simulink model "MMMS_v3"  (R2024b)
settings: Solver=VariableStepAuto  StartTime=0.0  StopTime=60  FixedStep=0.001  RelTol=1e-3
InitFcn:
  | %rho_0t=[0.29;0.29;0.29]; %m
  | %V_0t=[-0.001;-0.001;0];%[-0.0005;-0.0005;0];
  | %w_t=[0;0;-0.002];
  | 
  | 
  | %rho_0t=[0.3;0.3;0.2]; %m
  | %V_0t=[-0.001;-0.001;0];%[-0.0005;-0.0005;0];
  | %w_t=[0;0;-0.001];
values from neighbouring files (symbols this model uses):
  Dt = 0.1    [main_EKF.m]
  Fake_Manip_grad = -0.2.*eye(7)    [Initiate_FQ.m]
  g_cm = zeros(4,4,n)    [Initiate_KUKA_inv.m]    (also in Main_MMMS.m; test_KUKA_elements.m)
  g_It00 = [eye(3) rho_It;0 0 0 1]    [main_EKF.m]
  iota0 = eye(6,6)    [Initiate_KUKA_inv.m]    (also in Main_MMMS.m; test_KUKA_elements.m)
  K_d = 10*[1.3*eye(3) zeros(3);zeros(3) 0.8*eye(3)]    [Initiate_FQ.m]    (also in Initiate_KUKA_inv.m = 5*[0.7*eye(3) zeros(3);zeros(3) 0.5*eye(3)]; MMMS_Initiate_FQ.m; Main_MMMS.m = 5*[0.7*eye(3) zeros(3);zeros(3) 0.5*eye(3)]; test_KUKA_elements.m = 50*[0.7*eye(3) zeros(3);zeros(3) 0.5*eye(3)])
  K_i = 5*[0.1*eye(3) zeros(3);zeros(3) 0.01*eye(3)]    [Initiate_FQ.m]    (also in Initiate_KUKA_inv.m = 5*[0.01*eye(3) zeros(3);zeros(3) 0.001*eye(3)]; MMMS_Initiate_FQ.m; Main_MMMS.m = 5*[0.01*eye(3) zeros(3);zeros(3) 0.001*eye(3)]; test_KUKA_elements.m = 50*[0.01*eye(3) zeros(3);zeros(3) 0.001*eye(3)])
  K_p = 100*[0.1 0 0 0 0 0;0 0.1 0 0 0 0; 0 0 0.1 0 0 0; 0 0 0 0.01 0 0 ... (first row only)    [Initiate_FQ.m]    (also in Initiate_KUKA_inv.m = 5*[0.1 0 0 0 0 0;0 0.1 0 0 0 0; 0 0 0.1 0 0 0; 0 0 0 0.01 0 ; MMMS_Initiate_FQ.m; Main_MMMS.m = 5*[0.1 0 0 0 0 0;0 0.1 0 0 0 0; 0 0 0.1 0 0 0; 0 0 0 0.01 0 ; test_KUKA_elements.m = 50*[0.1 0 0 0 0 0;0 0.1 0 0 0 0; 0 0 0.1 0 0 0; 0 0 0 0.01 0)
  K_w = 200*eye(7)    [Initiate_FQ.m]    (also in MMMS_Initiate_FQ.m)
  K_wd = 2*eye(7)    [Initiate_FQ.m]    (also in MMMS_Initiate_FQ.m)
  m = randn(s,total_time_steps,6)*chol(R)    [main_EKF.m]
  M0 = M_temp.M0.data(:,:,1)    [Initiate_FQ.m]    (also in MMMS_Initiate_FQ.m; test_KUKA_elements.m)
  m0 = robot.Bodies{1,n+1}.Mass    [Initiate_KUKA_inv.m]    (also in Main_MMMS.m; test_KUKA_elements.m)
  m0_frak = diag_M(1:6,1:6)    [Initiate_KUKA_inv.m]    (also in Main_MMMS.m; make_uncertain.m = diag_M_unc(1:6,1:6); test_KUKA_elements.m)
  M0m = M_temp.M0m.data(:,:,1)    [Initiate_FQ.m]    (also in MMMS_Initiate_FQ.m; test_KUKA_elements.m)
  m_diag = diag_M(7:end,7:end)    [Initiate_KUKA_inv.m]    (also in Main_MMMS.m; make_uncertain.m = diag_M_unc(7:end,7:end); test_KUKA_elements.m)
  M_t = (((Adjoint(g_It))'\M_t_body)/(Adjoint(g_It)))    [Initiate_FQ.m]    (also in Initiate_KUKA_inv.m = [eye(3)*mt zeros(3); zeros(3) eye(3)*80]; MMMS_Initiate_FQ.m; Main_MMMS.m = [eye(3)*mt zeros(3); zeros(3) eye(3)*80]; test_KUKA_elements.m = [eye(3)*mt zeros(3); zeros(3) eye(3)*80])
  M_t_body = [eye(3)*mt zeros(3); zeros(3) eye(3)*0.416667]    [Initiate_FQ.m]    (also in MMMS_Initiate_FQ.m)
  mm = zeros(1,n)    [Initiate_KUKA_inv.m]    (also in Main_MMMS.m; test_KUKA_elements.m)
  mu = P0    [Initiate_FQ.m]    (also in Initiate_KUKA_inv.m = zeros(6,1); MMMS_Initiate_FQ.m; Main_MMMS.m = zeros(6,1); make_uncertain.m = P0_unc)
  mu_t = inv((Adjoint(g_It))')*M_t_body*[V_It;w_t]    [Initiate_FQ.m]    (also in Initiate_KUKA_inv.m = M_t*[V_0t;w_t]; MMMS_Initiate_FQ.m; Main_MMMS.m = M_t*[V_0t;w_t]; make_uncertain.m = inv((Adjoint(g_It))')*M_t_body_unc*[V_It;w_t])
  noise_st = 0.000005    (= 5e-06)    [main_EKF.m]
  q_dot_m = [0;0;0;0;0;0;0]    [Initiate_FQ.m]    (also in Initiate_KUKA_inv.m; MMMS_Initiate_FQ.m; Main_MMMS.m; test_KUKA_elements.m = [0])
  q_m = [0.2;1.2;0.3;2.5;0.5;1.5;0.6]    [Initiate_FQ.m]    (also in Initiate_KUKA_inv.m = [0;0;0;0;0;0;0]; MMMS_Initiate_FQ.m = [0.2;0.2;0.3;0.5;0.5;0.5;0.6]; Main_MMMS.m = [0;0;0;0;0;0;0]; test_KUKA_elements.m = [0.2;1.2;0.3;1.8;0.5;1.3;0.6])
  rho_It = [0;0;1.7]    [Initiate_FQ.m]    (also in MMMS_Initiate_FQ.m)
  s = RandStream.create('mrg32k3a','NumStreams',1)    [main_EKF.m]
  sc_size = 1    [Initiate_KUKA_inv.m]    (also in Main_MMMS.m; test_KUKA_elements.m)
  V_It = [0.0005;0.0005;0]    [Initiate_FQ.m]    (also in MMMS_Initiate_FQ.m = [0.001;0.001;0])
  Xi_m_matrix = zeros(6*n,n)    [Initiate_KUKA_inv.m]    (also in Main_MMMS.m)
undefined symbols (not defined in the file or in its folder): g_cm0, I0, Im, Mm, X, Xi_m, Y, Z
libraries: nesl_utility x314, sm_lib x231, robotcorelib x30, simulink x12
(part 3 of 13)

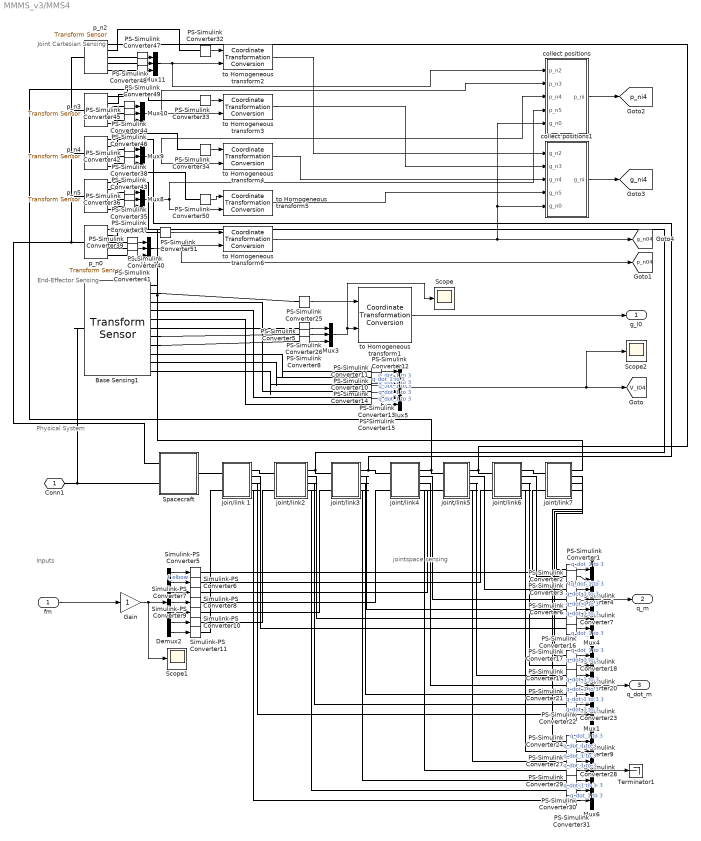
== system MMMS_v3/MMS4 ==
  note: Joint Cartesian Sensing
  note: End-Effector Sensing
  note: Inputs
  note: jointspace sensing
  note: Physical System
  fm : Inport
  Base Sensing1 : sm_lib/Frames and Transforms/Transform Sensor  MeasurementFrame=NonRotatingBase  RotationSequence=XYZ  SenseAngle=off  SenseAxis=off  SenseQ=off  SenseR=on  SenseRotationSequence=off  SenseOmegaX=on  SenseOmegaY=on  SenseOmegaZ=on  SenseOmega=off  SenseQDot=off  SenseRDot=off  SenseRotationSequenceDot=off  SenseAlphaX=off  SenseAlphaY=off  SenseAlphaZ=off  SenseAlpha=off  SenseQDDot=off  SenseRDDot=off  SenseX=on  SenseY=on  SenseZ=on  SenseXYZ=off  SenseRad=off  SenseAzim=off  SenseDist=off  SenseInc=off  SenseXDot=on  SenseYDot=on  SenseZDot=on  SenseXYZDot=off  SenseRadDot=off  SenseAzimDot=off  SenseDistDot=off  SenseIncDot=off  SenseXDDot=off  SenseYDDot=off  SenseZDDot=off  SenseXYZDDot=off  SenseRadDDot=off  SenseAzimDDot=off  SenseDistDDot=off  SenseIncDDot=off
  Demux2 : Demux  Outputs=7
  Gain : Gain
  Mux1 : Mux  Inputs=7
  Mux{2..3,8..11} (6 alike) : Mux  Inputs=3
  Mux4 : Mux  Inputs=7
  Mux5 : Mux  Inputs=6
  Mux6 : Mux  Inputs=7
  PS-Simulink Converter{1..51} (51 alike) : nesl_utility/PS-Simulink Converter  PhysicalDomain=network_engine_domain  SubClassName=ps_output  LeftPortType=input  RightPortType=output  PseudoPeriodic=off  Frequencies=[]  VectorFormat=1-D array  Unit=inherit  AffineConversion=off
  Scope : Scope
  Scope1 : Scope
  Scope2 : Scope
  Simulink-PS Converter{5..11} (7 alike) : nesl_utility/Simulink-PS Converter  PhysicalDomain=network_engine_domain  SubClassName=ps_input  LeftPortType=input  RightPortType=output  PseudoPeriodic=off  Frequencies=[]  NoiseDistribution=none  NoiseParameters=[]  Unit=1  AffineConversion=off  FilteringAndDerivatives=provide  SimscapeFilterOrder=1  InputFilterTimeConstant=0.001  UdotUserProvided=0
  Spacecraft : Subsystem
  Terminator1 : Terminator
  collect positions : MATLAB Function  TreatAsAtomicUnit=on
  collect positions1 : MATLAB Function  TreatAsAtomicUnit=on
  join/link 1 : Subsystem
  joint/link2 : Subsystem
  joint/link3 : Subsystem
  joint/link4 : Subsystem
  joint/link5 : Subsystem
  joint/link6 : Subsystem
  joint/link7 : Subsystem
  p_n{0,2..5} (5 alike) : sm_lib/Frames and Transforms/Transform Sensor  MeasurementFrame=Base  RotationSequence=XYZ  SenseAngle=off  SenseAxis=off  SenseQ=off  SenseR=on  SenseRotationSequence=off  SenseOmegaX=off  SenseOmegaY=off  SenseOmegaZ=off  SenseOmega=off  SenseQDot=off  SenseRDot=off  SenseRotationSequenceDot=off  SenseAlphaX=off  SenseAlphaY=off  SenseAlphaZ=off  SenseAlpha=off  SenseQDDot=off  SenseRDDot=off  SenseX=on  SenseY=on  SenseZ=on  SenseXYZ=off  SenseRad=off  SenseAzim=off  SenseDist=off  SenseInc=off  SenseXDot=off  SenseYDot=off  SenseZDot=off  SenseXYZDot=off  SenseRadDot=off  SenseAzimDot=off  SenseDistDot=off  SenseIncDot=off  SenseXDDot=off  SenseYDDot=off  SenseZDDot=off  SenseXYZDDot=off  SenseRadDDot=off  SenseAzimDDot=off  SenseDistDDot=off  SenseIncDDot=off
  to Homogeneous transform{1..6} (6 alike) : robotcorelib/Coordinate Transformation Conversion  InputRepresentation=Rotation Matrix  InputEulerSequence=ZYX  ShowTrVecInputPort=on  OutputRepresentation=Homogeneous Transformation  OutputEulerSequence=ZYX  ShowTrVecOutputPort=on  SimulateUsing=Code generation
  Conn1 : PMIOPort  Side=Left
  g_I0 : Outport
  q_m : Outport  Port=2
  q_dot_m : Outport  Port=3
  tag scope: V_I04=global, g_n04=global, g_ni4=global, p_n04=global, p_ni4=global
  wires:
  to Homogeneous transform5/1 -> collect positions1/4(g_n5)
  to Homogeneous transform4/1 -> collect positions1/3(g_n4)
  to Homogeneous transform3/1 -> collect positions1/2(g_n3)
  to Homogeneous transform2/1 -> collect positions1/1(g_n2)
  to Homogeneous transform6/1 -> [g_n04], collect positions1/5(g_n0), collect positions/5(g_n0)
  PS-Simulink Converter51/1 -> to Homogeneous transform6/1
  collect positions1/1(g_ni) -> [g_ni4]
  Mux8/1 -> collect positions/4(p_n5), to Homogeneous transform5/2
  PS-Simulink Converter50/1 -> to Homogeneous transform5/1
  PS-Simulink Converter34/1 -> to Homogeneous transform4/1
  Mux9/1 -> collect positions/3(p_n4), to Homogeneous transform4/2
  Mux10/1 -> collect positions/2(p_n3), to Homogeneous transform3/2
  PS-Simulink Converter33/1 -> to Homogeneous transform3/1
  PS-Simulink Converter32/1 -> to Homogeneous transform2/1
  collect positions/1(p_ni) -> [p_ni4]
  PS-Simulink Converter49/1 -> Mux11/3
  PS-Simulink Converter47/1 -> Mux11/1
  PS-Simulink Converter48/1 -> Mux11/2
  Mux11/1 -> collect positions/1(p_n2), to Homogeneous transform2/2
  PS-Simulink Converter46/1 -> Mux10/3
  PS-Simulink Converter44/1 -> Mux10/1
  PS-Simulink Converter45/1 -> Mux10/2
  PS-Simulink Converter43/1 -> Mux9/3
  PS-Simulink Converter38/1 -> Mux9/1
  PS-Simulink Converter42/1 -> Mux9/2
  PS-Simulink Converter37/1 -> Mux8/3
  PS-Simulink Converter35/1 -> Mux8/1
  PS-Simulink Converter36/1 -> Mux8/2
  PS-Simulink Converter41/1 -> Mux2/3
  PS-Simulink Converter40/1 -> Mux2/2
  PS-Simulink Converter39/1 -> Mux2/1
  Mux2/1 -> [p_n04], to Homogeneous transform6/2
  Mux5/1 -> Scope2/1, [V_I04]
  PS-Simulink Converter19/1 -> Mux1/3  "q_dot_1 to 3"
  PS-Simulink Converter17/1 -> Mux1/1  "q_dot_1 to 3"
  PS-Simulink Converter22/1 -> Mux1/6  "q_dot_1 to 3"
  PS-Simulink Converter29/1 -> Mux6/5  "q_dot_1 to 3"
  PS-Simulink Converter20/1 -> Mux1/4  "q_dot_1 to 3"
  Mux6/1 -> Terminator1/1
  PS-Simulink Converter24/1 -> Mux6/1  "q_dot_1 to 3"
  Mux1/1 -> q_dot_m/1
  Mux4/1 -> q_m/1
  PS-Simulink Converter28/1 -> Mux6/4  "q_dot_1 to 3"
  PS-Simulink Converter16/1 -> Mux4/7  "q_dot_1 to 3"
  PS-Simulink Converter23/1 -> Mux1/7  "q_dot_1 to 3"
  PS-Simulink Converter21/1 -> Mux1/5  "q_dot_1 to 3"
  PS-Simulink Converter4/1 -> Mux4/4  "q_dot_1 to 3"
  PS-Simulink Converter2/1 -> Mux4/2  "q_dot_1 to 3"
  PS-Simulink Converter7/1 -> Mux4/6  "q_dot_1 to 3"
  PS-Simulink Converter9/1 -> Mux6/2  "q_dot_1 to 3"
  PS-Simulink Converter31/1 -> Mux6/7  "q_dot_1 to 3"
  PS-Simulink Converter18/1 -> Mux1/2  "q_dot_1 to 3"
  PS-Simulink Converter3/1 -> Mux4/3  "q_dot_1 to 3"
  PS-Simulink Converter30/1 -> Mux6/6  "q_dot_1 to 3"
  PS-Simulink Converter6/1 -> Mux4/5  "q_dot_1 to 3"
  PS-Simulink Converter1/1 -> Mux4/1  "q_dot_1 to 3"
  PS-Simulink Converter27/1 -> Mux6/3  "q_dot_1 to 3"
  Demux2/5 -> Simulink-PS Converter9/1
  Demux2/2 -> Simulink-PS Converter6/1  "f_elbow"
  Demux2/6 -> Simulink-PS Converter10/1
  PS-Simulink Converter5/1 -> Mux3/2
  PS-Simulink Converter11/1 -> Mux5/1  "q_dot_1 to 3"
  Demux2/4 -> Simulink-PS Converter8/1
  PS-Simulink Converter14/1 -> Mux5/5  "q_dot_1 to 3"
  Demux2/7 -> Simulink-PS Converter11/1
  PS-Simulink Converter26/1 -> Mux3/1
  PS-Simulink Converter13/1 -> Mux5/4  "q_dot_1 to 3"
  to Homogeneous transform1/1 -> g_I0/1
  PS-Simulink Converter12/1 -> Mux5/2  "q_dot_1 to 3"
  Mux3/1 -> to Homogeneous transform1/2, Scope/1
  PS-Simulink Converter8/1 -> Mux3/3
  Gain/1 -> Demux2/1, Scope1/1
  PS-Simulink Converter25/1 -> to Homogeneous transform1/1
  fm/1 -> Gain/1
  PS-Simulink Converter10/1 -> Mux5/3  "q_dot_1 to 3"
  PS-Simulink Converter15/1 -> Mux5/6  "q_dot_1 to 3"
  Demux2/3 -> Simulink-PS Converter7/1
  Demux2/1 -> Simulink-PS Converter5/1
  connections:
  p_n0/RConn2 -- PS-Simulink Converter51/LConn1
  p_n5/RConn2 -- PS-Simulink Converter50/LConn1
  p_n4/RConn2 -- PS-Simulink Converter34/LConn1
  p_n3/RConn2 -- PS-Simulink Converter33/LConn1
  PS-Simulink Converter32/LConn1 -- p_n2/RConn2
  p_n2/RConn4 -- PS-Simulink Converter48/LConn1
  p_n2/RConn3 -- PS-Simulink Converter47/LConn1
  PS-Simulink Converter49/LConn1 -- p_n2/RConn5
  p_n3/RConn4 -- PS-Simulink Converter45/LConn1
  p_n3/RConn3 -- PS-Simulink Converter44/LConn1
  PS-Simulink Converter46/LConn1 -- p_n3/RConn5
  p_n4/RConn4 -- PS-Simulink Converter42/LConn1
  p_n4/RConn3 -- PS-Simulink Converter38/LConn1
  PS-Simulink Converter43/LConn1 -- p_n4/RConn5
  p_n5/RConn4 -- PS-Simulink Converter36/LConn1
  p_n5/RConn3 -- PS-Simulink Converter35/LConn1
  PS-Simulink Converter37/LConn1 -- p_n5/RConn5
  p_n0/RConn3 -- PS-Simulink Converter39/LConn1
  p_n0/LConn1 -- p_n5/LConn1 -- p_n4/LConn1 -- p_n3/LConn1 -- p_n2/LConn1 -- Spacecraft/LConn1
  p_n0/RConn4 -- PS-Simulink Converter40/LConn1
  PS-Simulink Converter41/LConn1 -- p_n0/RConn5
  join/link 1/RConn3 -- PS-Simulink Converter23/LConn1
  joint/link2/RConn3 -- PS-Simulink Converter22/LConn1
  join/link 1/RConn4 -- PS-Simulink Converter31/LConn1
  joint/link2/RConn4 -- PS-Simulink Converter30/LConn1
  PS-Simulink Converter7/LConn1 -- joint/link2/RConn2
  join/link 1/RConn2 -- PS-Simulink Converter16/LConn1
  joint/link2/RConn1 -- p_n5/RConn1 -- joint/link3/LConn1
  Simulink-PS Converter10/RConn1 -- joint/link2/LConn2
  join/link 1/RConn1 -- joint/link2/LConn1
  join/link 1/LConn1 -- Spacecraft/RConn1
  join/link 1/LConn2 -- Simulink-PS Converter11/RConn1
  joint/link7/RConn4 -- PS-Simulink Converter24/LConn1
  joint/link7/RConn3 -- PS-Simulink Converter17/LConn1
  joint/link7/RConn2 -- PS-Simulink Converter1/LConn1
  joint/link6/LConn2 -- Simulink-PS Converter6/RConn1
  joint/link6/RConn2 -- PS-Simulink Converter2/LConn1
  joint/link6/RConn1 -- joint/link7/LConn1
  joint/link3/RConn4 -- PS-Simulink Converter29/LConn1
  joint/link3/RConn3 -- PS-Simulink Converter21/LConn1
  joint/link3/RConn2 -- PS-Simulink Converter6/LConn1
  joint/link4/RConn4 -- PS-Simulink Converter28/LConn1
  joint/link4/RConn3 -- PS-Simulink Converter20/LConn1
  joint/link4/RConn2 -- PS-Simulink Converter4/LConn1
  joint/link5/RConn4 -- PS-Simulink Converter27/LConn1
  joint/link5/RConn3 -- PS-Simulink Converter19/LConn1
  joint/link5/RConn2 -- PS-Simulink Converter3/LConn1
  joint/link6/RConn4 -- PS-Simulink Converter9/LConn1
  joint/link6/RConn3 -- PS-Simulink Converter18/LConn1
  Simulink-PS Converter7/RConn1 -- joint/link5/LConn2
  Base Sensing1/RConn6 -- PS-Simulink Converter26/LConn1
  Base Sensing1/RConn8 -- PS-Simulink Converter8/LConn1
  Base Sensing1/RConn9 -- PS-Simulink Converter11/LConn1
  Base Sensing1/RConn4 -- PS-Simulink Converter14/LConn1
  Simulink-PS Converter5/RConn1 -- joint/link7/LConn2
  Base Sensing1/RConn3 -- PS-Simulink Converter13/LConn1
  Base Sensing1/RConn11 -- PS-Simulink Converter10/LConn1
  p_n2/RConn1 -- joint/link5/RConn1 -- joint/link6/LConn1
  Base Sensing1/RConn7 -- PS-Simulink Converter5/LConn1
  Base Sensing1/RConn5 -- PS-Simulink Converter15/LConn1
  p_n3/RConn1 -- joint/link4/RConn1 -- joint/link5/LConn1
  Base Sensing1/RConn2 -- PS-Simulink Converter25/LConn1
  Simulink-PS Converter8/RConn1 -- joint/link4/LConn2
  Simulink-PS Converter9/RConn1 -- joint/link3/LConn2
  Base Sensing1/RConn10 -- PS-Simulink Converter12/LConn1
  joint/link3/RConn1 -- p_n4/RConn1 -- joint/link4/LConn1
  joint/link7/RConn1 -- Base Sensing1/RConn1 -- p_n0/RConn1
  Base Sensing1/LConn1 -- Spacecraft/LConn2 -- Conn1/RConn1

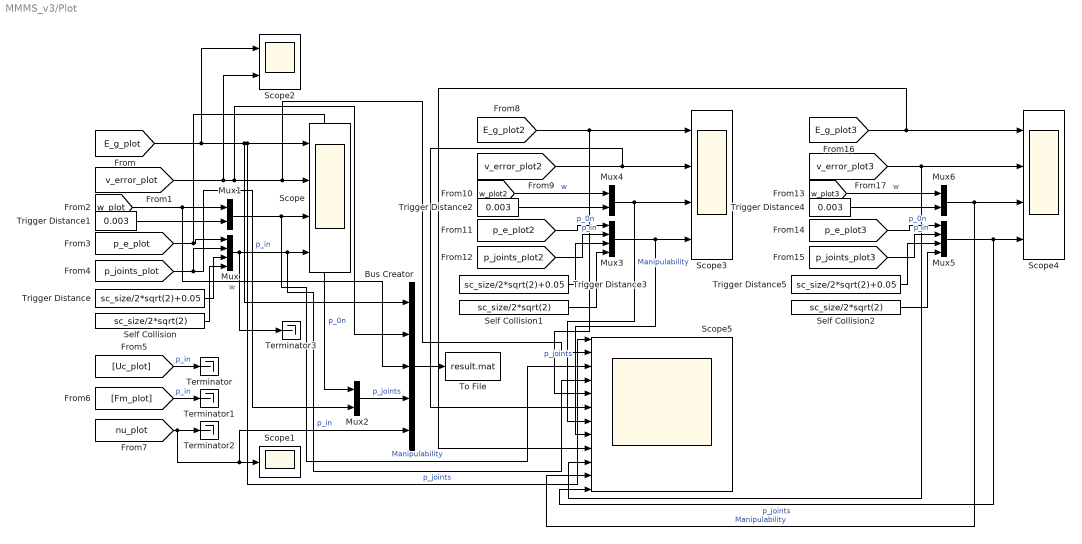
== system MMMS_v3/Plot ==
  Bus Creator : BusCreator  Inputs=5
  Mux : Mux  Inputs=[1 4 1 1]
  Mux{1..2,4,6} (4 alike) : Mux  Inputs=2
  Mux3 : Mux  Inputs=[1 4 1 1]
  Mux5 : Mux  Inputs=[1 4 1 1]
  Scope : Scope  NumInputPorts=4
  Scope1 : Scope
  Scope2 : Scope  NumInputPorts=2
  Scope3 : Scope  NumInputPorts=4
  Scope4 : Scope  NumInputPorts=4
  Scope5 : Scope  NumInputPorts=12
  Self Collision : Constant  Value=sc_size/2*sqrt(2)
  Self Collision1 : Constant  Value=sc_size/2*sqrt(2)
  Self Collision2 : Constant  Value=sc_size/2*sqrt(2)
  Terminator{,1..3} (4 alike) : Terminator
  To File : ToFile  Filename=result.mat
  Trigger Distance : Constant  Value=sc_size/2*sqrt(2)+0.05
  Trigger Distance1 : Constant  Value=0.003
  Trigger Distance2 : Constant  Value=0.003
  Trigger Distance3 : Constant  Value=sc_size/2*sqrt(2)+0.05
  Trigger Distance4 : Constant  Value=0.003
  Trigger Distance5 : Constant  Value=sc_size/2*sqrt(2)+0.05
  wires:
  [E_g_plot] -> Scope2/1, Bus Creator/1, Scope/1, Scope5/1
  [v_error_plot] -> Scope2/2, Bus Creator/2, Scope5/2, Scope/2
  [w_plot] -> Bus Creator/3, Mux1/1  "w"
  [p_e_plot] -> Mux2/1, Mux/1  "p_0n"
  [p_joints_plot] -> Mux/2, Mux2/2  "p_in"
  Mux/1 -> Scope5/4, Scope/4, Terminator3/1  "p_joints"
  Trigger Distance/1 -> Mux/3
  [Uc_plot] -> Terminator/1  "p_in"
  [Fm_plot] -> Terminator1/1  "p_in"
  [nu_plot] -> Bus Creator/5, Scope1/1, Terminator2/1  "p_in"
  Self Collision/1 -> Mux/4
  Trigger Distance1/1 -> Mux1/2
  Mux1/1 -> Scope5/3, Scope/3  "Manipulability"
  Bus Creator/1 -> To File/1
  Mux2/1 -> Bus Creator/4  "p_joints"
  [w_plot2] -> Mux4/1  "w"
  [v_error_plot2] -> Scope5/6, Scope3/2
  [p_joints_plot2] -> Mux3/2  "p_in"
  [E_g_plot2] -> Scope5/5, Scope3/1
  Trigger Distance2/1 -> Mux4/2
  Mux3/1 -> Scope5/8, Scope3/4  "p_joints"
  [p_e_plot2] -> Mux3/1  "p_0n"
  Mux4/1 -> Scope5/7, Scope3/3  "Manipulability"
  Trigger Distance3/1 -> Mux3/3
  Self Collision1/1 -> Mux3/4
  [p_joints_plot3] -> Mux5/2  "p_in"
  Trigger Distance5/1 -> Mux5/3
  Mux6/1 -> Scope5/11, Scope4/3  "Manipulability"
  Trigger Distance4/1 -> Mux6/2
  Mux5/1 -> Scope5/12, Scope4/4  "p_joints"
  [v_error_plot3] -> Scope5/10, Scope4/2
  [E_g_plot3] -> Scope5/9, Scope4/1
  [p_e_plot3] -> Mux5/1  "p_0n"
  Self Collision2/1 -> Mux5/4
  [w_plot3] -> Mux6/1  "w"

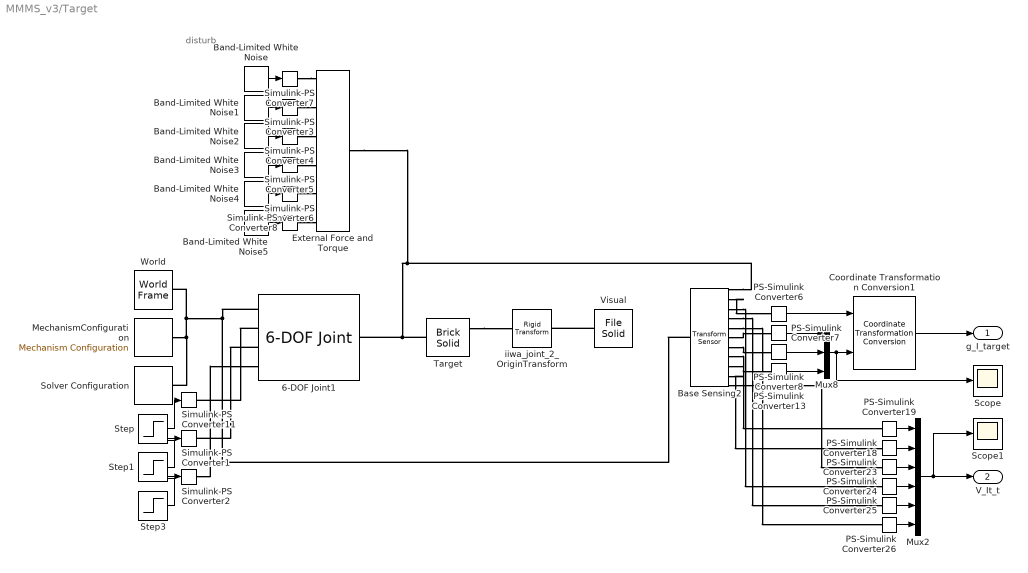
== system MMMS_v3/Target ==
  note: disturb
  6-DOF Joint1 : sm_lib/Joints/6-DOF Joint  JointMode=Normal  CompositeWrenchDir=FollowerOnBase  CompositeWrenchFrame=BaseFrame  SenseConstraintForce=off  SenseConstraintTorque=off  SenseTotalForce=off  SenseTotalTorque=off  PxPositionTargetSpecify=on  PxPositionTargetPriority=High  PxPositionTargetValue=rho_It(1)  PxPositionTargetValueUnits=m  PxVelocityTargetSpecify=on  PxVelocityTargetPriority=High  PxVelocityTargetValue=V_It(1)  PxVelocityTargetValueUnits=m/s  PxEquilibriumPosition=0  PxEquilibriumPositionUnits=m  PxSpringStiffness=0  PxSpringStiffnessUnits=N/m  PxDampingCoefficient=0  PxDampingCoefficientUnits=N/(m/s)  PxLowerLimitSpecify=off  PxLowerLimitBound=-1  PxLowerLimitBoundUnits=m  PxLowerLimitStiffness=1e6  PxLowerLimitStiffnessUnits=N/m  PxLowerLimitDamping=1e3  PxLowerLimitDampingUnits=N/(m/s)  PxLowerLimitTransitionRegionWidth=1e-4  PxLowerLimitTransitionRegionWidthUnits=m  PxUpperLimitSpecify=off  PxUpperLimitBound=1  PxUpperLimitBoundUnits=m  PxUpperLimitStiffness=1e6  PxUpperLimitStiffnessUnits=N/m  PxUpperLimitDamping=1e3  PxUpperLimitDampingUnits=N/(m/s)  PxUpperLimitTransitionRegionWidth=1e-4  PxUpperLimitTransitionRegionWidthUnits=m  PxTorqueActuationMode=InputTorque  PxMotionActuationMode=ComputedMotion  PxSensePosition=off  PxSenseVelocity=off  PxSenseAcceleration=off  PxSenseTorqueForce=off  PxSenseLowerLimitTorqueForce=off  PxSenseUpperLimitTorqueForce=off  PyPositionTargetSpecify=on  PyPositionTargetPriority=High  PyPositionTargetValue=rho_It(2)  PyPositionTargetValueUnits=m  PyVelocityTargetSpecify=on  PyVelocityTargetPriority=High  PyVelocityTargetValue=V_It(2)  PyVelocityTargetValueUnits=m/s  PyEquilibriumPosition=0  PyEquilibriumPositionUnits=m  PySpringStiffness=0  PySpringStiffnessUnits=N/m  PyDampingCoefficient=0  PyDampingCoefficientUnits=N/(m/s)  PyLowerLimitSpecify=off  PyLowerLimitBound=-1  PyLowerLimitBoundUnits=m  PyLowerLimitStiffness=1e6  PyLowerLimitStiffnessUnits=N/m  PyLowerLimitDamping=1e3  PyLowerLimitDampingUnits=N/(m/s)  PyLowerLimitTransitionRegionWidth=1e-4  PyLowerLimitTransitionRegionWidthUnits=m  PyUpperLimitSpecify=off  PyUpperLimitBound=1  PyUpperLimitBoundUnits=m  PyUpperLimitStiffness=1e6  PyUpperLimitStiffnessUnits=N/m  PyUpperLimitDamping=1e3  PyUpperLimitDampingUnits=N/(m/s)  PyUpperLimitTransitionRegionWidth=1e-4  PyUpperLimitTransitionRegionWidthUnits=m  PyTorqueActuationMode=InputTorque  PyMotionActuationMode=ComputedMotion  PySensePosition=off  PySenseVelocity=off  PySenseAcceleration=off  PySenseTorqueForce=off  PySenseLowerLimitTorqueForce=off  PySenseUpperLimitTorqueForce=off  PzPositionTargetSpecify=on  PzPositionTargetPriority=High  PzPositionTargetValue=rho_It(3)  PzPositionTargetValueUnits=m  PzVelocityTargetSpecify=on  PzVelocityTargetPriority=High  PzVelocityTargetValue=V_It(3)  PzVelocityTargetValueUnits=m/s  PzEquilibriumPosition=0  PzEquilibriumPositionUnits=m  PzSpringStiffness=0  PzSpringStiffnessUnits=N/m  PzDampingCoefficient=0  PzDampingCoefficientUnits=N/(m/s)  PzLowerLimitSpecify=off  PzLowerLimitBound=-1  PzLowerLimitBoundUnits=m  PzLowerLimitStiffness=1e6  PzLowerLimitStiffnessUnits=N/m  PzLowerLimitDamping=1e3  PzLowerLimitDampingUnits=N/(m/s)  PzLowerLimitTransitionRegionWidth=1e-4  PzLowerLimitTransitionRegionWidthUnits=m  PzUpperLimitSpecify=off  PzUpperLimitBound=1  PzUpperLimitBoundUnits=m  PzUpperLimitStiffness=1e6  PzUpperLimitStiffnessUnits=N/m  PzUpperLimitDamping=1e3  PzUpperLimitDampingUnits=N/(m/s)  PzUpperLimitTransitionRegionWidth=1e-4  PzUpperLimitTransitionRegionWidthUnits=m  PzTorqueActuationMode=InputTorque  PzMotionActuationMode=ComputedMotion  PzSensePosition=off  PzSenseVelocity=off  PzSenseAcceleration=off  PzSenseTorqueForce=off  PzSenseLowerLimitTorqueForce=off  PzSenseUpperLimitTorqueForce=off  SphPositionTargetSpecify=on  SphPositionTargetPriority=High  SphPositionTargetRotationMethod=RotationSequence  SphPositionTargetFollAlignAxisA=+X  SphPositionTargetBaseAlignAxisA=+Y  SphPositionTargetFollAlignAxisB=+Y  SphPositionTargetBaseAlignAxisB=+Z  SphPositionTargetRotationStandardAxis=+Z  SphPositionTargetRotationAngle=0.0  SphPositionTargetRotationAngleUnits=deg  SphPositionTargetRotationArbitraryAxis=[0 0 1]  SphPositionTargetRotationSequenceAxes=FollowerAxes  SphPositionTargetRotationSequence=XYZ  SphPositionTargetRotationSequenceAngles=[0 0 0]  SphPositionTargetRotationSequenceAnglesUnits=rad  SphPositionTargetRotationMatrix=[1 0 0; 0 1 0; 0 0 1]  SphPositionTargetQuaternion=[1 0 0 0]  SphVelocityTargetSpecify=on  SphVelocityTargetPriority=High  SphVelocityTargetValue=w_t  SphVelocityTargetValueUnits=rad/s  SphVelocityTargetInFollowerFrame=off  SphEqPosRotationMethod=None  SphEqPosFollAlignAxisA=+X  SphEqPosBaseAlignAxisA=+Y  SphEqPosFollAlignAxisB=+Y  SphEqPosBaseAlignAxisB=+Z  SphEqPosRotationStandardAxis=+Z  SphEqPosRotationAngle=0.0  SphEqPosRotationAngleUnits=deg  SphEqPosRotationArbitraryAxis=[0 0 1]  SphEqPosRotationSequenceAxes=FollowerAxes  SphEqPosRotationSequence=XYX  SphEqPosRotationSequenceAngles=[0 0 0]  SphEqPosRotationSequenceAnglesUnits=deg  SphEqPosRotationMatrix=[1 0 0; 0 1 0; 0 0 1]  SphEqPosQuaternion=[1 0 0 0]  SphSpringStiffness=0  SphSpringStiffnessUnits=N*m/deg  SphDampingCoefficient=0  SphDampingCoefficientUnits=N*m/(deg/s)  SphLowerLimitSpecify=off  SphLowerLimitBound=15  SphLowerLimitBoundUnits=deg  SphLowerLimitStiffness=1e4  SphLowerLimitStiffnessUnits=N*m/deg  SphLowerLimitDamping=10  SphLowerLimitDampingUnits=N*m/(deg/s)  SphLowerLimitTransitionRegionWidth=0.1  SphLowerLimitTransitionRegionWidthUnits=deg  SphUpperLimitSpecify=off  SphUpperLimitBound=45  SphUpperLimitBoundUnits=deg  SphUpperLimitStiffness=1e4  SphUpperLimitStiffnessUnits=N*m/deg  SphUpperLimitDamping=10  SphUpperLimitDampingUnits=N*m/(deg/s)  SphUpperLimitTransitionRegionWidth=0.1  SphUpperLimitTransitionRegionWidthUnits=deg  SphTorqueActuationMode=NoTorque  SphActuateTorqueX=off  SphActuateTorqueY=off  SphActuateTorqueZ=off  SphActuateTorque=off  SphActuationFrame=BaseFrame  SphSensePosition=off  SphSenseVelocityX=off  SphSenseVelocityY=off  SphSenseVelocityZ=off  SphSenseVelocity=off  SphSenseAccelerationX=off  SphSenseAccelerationY=off  SphSenseAccelerationZ=off  SphSenseAcceleration=off  SphSenseLowerLimitTorqueMag=off  SphSenseUpperLimitTorqueMag=off  SphSensingFrame=BaseFrame
  Band-Limited White Noise : simulink/Sources/Band-Limited White Noise  Cov=dist_force  Ts=0.1  seed=[23347]
  Band-Limited White Noise1 : simulink/Sources/Band-Limited White Noise  Cov=dist_force  Ts=0.1  seed=[23348]
  Band-Limited White Noise2 : simulink/Sources/Band-Limited White Noise  Cov=[0.0000001]  Ts=0.1  seed=[23343]
  Band-Limited White Noise3 : simulink/Sources/Band-Limited White Noise  Cov=dist_force  Ts=0.1  seed=[23342]
  Band-Limited White Noise4 : simulink/Sources/Band-Limited White Noise  Cov=dist_Force  Ts=0.1  seed=[23345]
  Band-Limited White Noise5 : simulink/Sources/Band-Limited White Noise  Cov=dist_force  Ts=0.1  seed=[23341]
  Base Sensing2 : sm_lib/Frames and Transforms/Transform Sensor  MeasurementFrame=NonRotatingBase  RotationSequence=XYZ  SenseAngle=off  SenseAxis=off  SenseQ=off  SenseR=on  SenseRotationSequence=off  SenseOmegaX=on  SenseOmegaY=on  SenseOmegaZ=on  SenseOmega=off  SenseQDot=off  SenseRDot=off  SenseRotationSequenceDot=off  SenseAlphaX=off  SenseAlphaY=off  SenseAlphaZ=off  SenseAlpha=off  SenseQDDot=off  SenseRDDot=off  SenseX=on  SenseY=on  SenseZ=on  SenseXYZ=off  SenseRad=off  SenseAzim=off  SenseDist=off  SenseInc=off  SenseXDot=on  SenseYDot=on  SenseZDot=on  SenseXYZDot=off  SenseRadDot=off  SenseAzimDot=off  SenseDistDot=off  SenseIncDot=off  SenseXDDot=off  SenseYDDot=off  SenseZDDot=off  SenseXYZDDot=off  SenseRadDDot=off  SenseAzimDDot=off  SenseDistDDot=off  SenseIncDDot=off
  Coordinate Transformation Conversion1 : robotcorelib/Coordinate Transformation Conversion  InputRepresentation=Rotation Matrix  InputEulerSequence=ZYX  ShowTrVecInputPort=on  OutputRepresentation=Homogeneous Transformation  OutputEulerSequence=ZYX  ShowTrVecOutputPort=on  SimulateUsing=Interpreted execution
  External Force and Torque : sm_lib/Forces and Torques/External Force and Torque  EnableForceX=on  EnableForceY=on  EnableForceZ=on  EnableForce=off  ForceResolutionFrame=AttachedFrame  EnableTorqueX=on  EnableTorqueY=on  EnableTorqueZ=on  EnableTorque=off  TorqueResolutionFrame=AttachedFrame
  MechanismConfiguration : sm_lib/Utilities/Mechanism Configuration  UniformGravity=Constant  GravityVector=[0 0 0]  GravityVectorUnits=m/s^2  LinearizationDelta=0.001  JointModeTransitionNonlinearIterations=2
  Mux2 : Mux  Inputs=6
  Mux8 : Mux  Inputs=3
  PS-Simulink Converter{6..8,13,18..19,23..26} (10 alike) : nesl_utility/PS-Simulink Converter  PhysicalDomain=network_engine_domain  SubClassName=ps_output  LeftPortType=input  RightPortType=output  PseudoPeriodic=off  Frequencies=[]  VectorFormat=1-D array  Unit=inherit  AffineConversion=off
  Scope : Scope
  Scope1 : Scope
  Simulink-PS Converter{1..8,11} (9 alike) : nesl_utility/Simulink-PS Converter  PhysicalDomain=network_engine_domain  SubClassName=ps_input  LeftPortType=input  RightPortType=output  PseudoPeriodic=off  Frequencies=[]  NoiseDistribution=none  NoiseParameters=[]  Unit=1  AffineConversion=off  FilteringAndDerivatives=provide  SimscapeFilterOrder=1  InputFilterTimeConstant=0.001  UdotUserProvided=0
  Solver Configuration : nesl_utility/Solver Configuration  PhysicalDomain=network_engine_domain  SubClassName=solver  LeftPortType=input  RightPortType=generic  Tones=[]  Harmonics=[]  SimulateNoise=off  Profile=off  UseLocalSampling=off  EnableSwitchedLinearOptims=on  FrequencyDomain=off  UseCCode=off  RelTol=0.001  AbsTol=0.001  MinStep=1e-09  ToWorkspace=off  RevertToSquareIcSolve=off  NumHomotopyIterations=100  PhasorMode=off  PhasorModeNumHarmonics=1  ConsistencySolver=NEWTON_FTOL  IndexReductionMethod=DerivativeReplacement  DoDC=off  ResidualTolerance=1e-09  ConsistencyTolSource=GLOBAL  ConsistencyAbsTol=0.001  ConsistencyRelTol=0.001  ConsistencyTolFactor=0.001  UseLocalSolver=off  LocalSolverChoice=NE_BACKWARD_EULER_ADVANCER  ResolveIndetEquations=on  FunctionEvalNumThread=1  LocalSolverSampleTime=0.001  DoFixedCost=off  MaxNonlinIter=3  MaxModeIter=2  ComputeImpulses=off  ImpulseIterations=2  LinearAlgebra=Full  LinearAlgebraNumThread=0  EquationFormulation=NE_TIME_EF  DelaysMemoryBudget=1024  AutomaticFiltering=on  FilteringTimeConstant=0.001  PartitionStorageMethod=AS_NEEDED  PartitionMemoryBudget=1024  PartitionMethod=ROBUST  MultibodyUseLocalSolver=off  MultibodyLocalSolverChoice=ODE1  MultibodyLocalSolverSampleTime=0.001
  Step : Step  Time=50  After=-0.004  SampleTime=0
  Step1 : Step  Time=50  After=-0.004  SampleTime=0
  Step3 : Step  Time=50  After=-0.0002  SampleTime=0
  Target : sm_lib/Body Elements/Brick Solid  BrickDimensions=[0.5, 0.5, 0.5]  BrickDimensionsUnits=m  ExportEntireGeometry=on  InertiaType=Custom  BasedOnType=Mass  Density=1000  DensityUnits=kg/m^3  Mass=10  MassUnits=kg  CenterOfMass=[0 0 0]  CenterOfMassUnits=m  MomentsOfInertia=[M_t(4,4) M_t(5,5) M_t(6,6)]  MomentsOfInertiaUnits=kg*m^2  ProductsOfInertia=[0 0 0]  ProductsOfInertiaUnits=kg*m^2  GraphicType=None  MarkerShape=Sphere  MarkerSize=10  GraphicVisPropType=SimpleVisualProperties  GraphicDiffuseColor=[0.5 0.5 0.5]  GraphicOpacity=1.0  GraphicSpecularColor=[0.5 0.5 0.5 1.0]  GraphicAmbientColor=[0.15 0.15 0.15 1.0]  GraphicEmissiveColor=[0.0 0.0 0.0 1.0]  GraphicShininess=75  DoExposeReferenceFrame=on  SerializedFrames=<Frames><Frame><Id>Frame1</Id><Value><Name>F1</Name><Origin><Source>GeometricFeature</Source><FeatureName>-x -y -z point</FeatureName></Origin><PrimaryAxis><DefinedDirection>+Z</DefinedDirection><Source>ReferenceFrame</Source><SourceDirection>+Z</SourceDirection><FeatureName></FeatureName></PrimaryAxis><SecondaryAxis><DefinedDirection>+X</DefinedDirection><Source>ReferenceFrame</Source><SourceDirection>+X</SourceDirection><FeatureName></FeatureName></SecondaryAxis></Value></Frame></Frames>
  Visual : sm_lib/Body Elements/File Solid  ExtGeomFileName=Spacecrafts/CubeSatAssembly_wo_antennas.stl  UnitType=Custom  ExtGeomFileUnits=cm  StepReaderType=HEX  ExportConvexHullGeometry=off  InertiaType=Custom  BasedOnType=DensityFromFile  Density=1000  DensityUnits=kg/m^3  Mass=0  MassUnits=kg  CenterOfMass=[0, 0, 0]  CenterOfMassUnits=m  MomentsOfInertia=[0, 0, 0]  MomentsOfInertiaUnits=kg*m^2  ProductsOfInertia=[0, 0, 0]  ProductsOfInertiaUnits=kg*m^2  GraphicType=FromGeometry  MarkerShape=Sphere  MarkerSize=10  GraphicVisPropType=SimpleVisualProperties  GraphicDiffuseColor=[0.7 0.7 0.7]  GraphicOpacity=1  GraphicSpecularColor=[0.5 0.5 0.5 1.0]  GraphicAmbientColor=[0.15 0.15 0.15 1.0]  GraphicEmissiveColor=[0.0 0.0 0.0 1.0]  GraphicShininess=75  DoExposeReferenceFrame=on  SerializedFrames=<Frames/>
  World : sm_lib/Frames and Transforms/World Frame
  iiwa_joint_2_OriginTransform : sm_lib/Frames and Transforms/Rigid Transform  RotationMethod=RotationSequence  FollAlignAxisA=+X  BaseAlignAxisA=+Y  FollAlignAxisB=+Y  BaseAlignAxisB=+Z  RotationStandardAxis=+Z  RotationAngle=0.0  RotationAngleUnits=deg  RotationArbitraryAxis=[0 0 1]  RotationSequenceAxes=FollowerAxes  RotationSequence=XYZ  RotationSequenceAngles=[0 0 0]  RotationSequenceAnglesUnits=rad  RotationMatrix=[1 0 0; 0 1 0; 0 0 1]  Quaternion=[1 0 0 0]  TranslationMethod=Cartesian  TranslationCartesianOffset=[-3.28, -4.43, 0.817]+[0.25, 0.25, 0.25]  TranslationCartesianOffsetUnits=m  TranslationStandardAxis=+Z  TranslationStandardOffset=0  TranslationStandardOffsetUnits=m  TranslationROffset=0  TranslationROffsetUnits=m  TranslationThetaOffset=0  TranslationThetaOffsetUnits=deg  TranslationZOffset=0  TranslationZOffsetUnits=m
  g_I_target : Outport
  V_It_t : Outport  Port=2
  wires:
  PS-Simulink Converter13/1 -> Mux8/3
  Coordinate Transformation Conversion1/1 -> g_I_target/1
  PS-Simulink Converter7/1 -> Mux8/1
  PS-Simulink Converter6/1 -> Coordinate Transformation Conversion1/1
  PS-Simulink Converter8/1 -> Mux8/2
  Mux8/1 -> Scope/1, Coordinate Transformation Conversion1/2
  PS-Simulink Converter24/1 -> Mux2/4
  PS-Simulink Converter18/1 -> Mux2/2
  PS-Simulink Converter25/1 -> Mux2/5
  Mux2/1 -> Scope1/1, V_It_t/1
  PS-Simulink Converter19/1 -> Mux2/1
  PS-Simulink Converter23/1 -> Mux2/3
  PS-Simulink Converter26/1 -> Mux2/6
  Step/1 -> Simulink-PS Converter11/1
  Step1/1 -> Simulink-PS Converter1/1
  Step3/1 -> Simulink-PS Converter2/1
  Band-Limited White Noise2/1 -> Simulink-PS Converter4/1
  Band-Limited White Noise4/1 -> Simulink-PS Converter6/1
  Band-Limited White Noise5/1 -> Simulink-PS Converter8/1
  Band-Limited White Noise3/1 -> Simulink-PS Converter5/1
  Band-Limited White Noise1/1 -> Simulink-PS Converter3/1
  Band-Limited White Noise/1 -> Simulink-PS Converter7/1
  connections:
  Target/RConn1 -- External Force and Torque/RConn1 -- Base Sensing2/RConn1 -- 6-DOF Joint1/RConn1
  Base Sensing2/RConn2 -- PS-Simulink Converter6/LConn1
  Base Sensing2/RConn3 -- PS-Simulink Converter24/LConn1
  World/RConn1 -- MechanismConfiguration/RConn1 -- Solver Configuration/RConn1 -- 6-DOF Joint1/LConn1 -- Base Sensing2/LConn1
  Base Sensing2/RConn5 -- PS-Simulink Converter26/LConn1
  Visual/RConn1 -- iiwa_joint_2_OriginTransform/RConn1
  Base Sensing2/RConn4 -- PS-Simulink Converter25/LConn1
  Base Sensing2/RConn6 -- PS-Simulink Converter7/LConn1
  Base Sensing2/RConn7 -- PS-Simulink Converter8/LConn1
  Base Sensing2/RConn8 -- PS-Simulink Converter13/LConn1
  Base Sensing2/RConn9 -- PS-Simulink Converter19/LConn1
  Base Sensing2/RConn10 -- PS-Simulink Converter18/LConn1
  Base Sensing2/RConn11 -- PS-Simulink Converter23/LConn1
  Target/LConn1 -- iiwa_joint_2_OriginTransform/LConn1
  6-DOF Joint1/LConn2 -- Simulink-PS Converter11/RConn1
  6-DOF Joint1/LConn3 -- Simulink-PS Converter1/RConn1
  Simulink-PS Converter2/RConn1 -- 6-DOF Joint1/LConn4
  Simulink-PS Converter6/RConn1 -- External Force and Torque/LConn5
  Simulink-PS Converter3/RConn1 -- External Force and Torque/LConn2
  Simulink-PS Converter7/RConn1 -- External Force and Torque/LConn1
  Simulink-PS Converter8/RConn1 -- External Force and Torque/LConn6
  Simulink-PS Converter5/RConn1 -- External Force and Torque/LConn4
  Simulink-PS Converter4/RConn1 -- External Force and Torque/LConn3

== system MMMS_v3/Target1 ==
  6-DOF Joint1 : sm_lib/Joints/6-DOF Joint  JointMode=Disengaged  CompositeWrenchDir=FollowerOnBase  CompositeWrenchFrame=BaseFrame  SenseConstraintForce=off  SenseConstraintTorque=off  SenseTotalForce=off  SenseTotalTorque=off  PxPositionTargetSpecify=on  PxPositionTargetPriority=High  PxPositionTargetValue=rho_It(1)  PxPositionTargetValueUnits=m  PxVelocityTargetSpecify=on  PxVelocityTargetPriority=High  PxVelocityTargetValue=V_It(1)  PxVelocityTargetValueUnits=m/s  PxEquilibriumPosition=0  PxEquilibriumPositionUnits=m  PxSpringStiffness=0  PxSpringStiffnessUnits=N/m  PxDampingCoefficient=0  PxDampingCoefficientUnits=N/(m/s)  PxLowerLimitSpecify=off  PxLowerLimitBound=-1  PxLowerLimitBoundUnits=m  PxLowerLimitStiffness=1e6  PxLowerLimitStiffnessUnits=N/m  PxLowerLimitDamping=1e3  PxLowerLimitDampingUnits=N/(m/s)  PxLowerLimitTransitionRegionWidth=1e-4  PxLowerLimitTransitionRegionWidthUnits=m  PxUpperLimitSpecify=off  PxUpperLimitBound=1  PxUpperLimitBoundUnits=m  PxUpperLimitStiffness=1e6  PxUpperLimitStiffnessUnits=N/m  PxUpperLimitDamping=1e3  PxUpperLimitDampingUnits=N/(m/s)  PxUpperLimitTransitionRegionWidth=1e-4  PxUpperLimitTransitionRegionWidthUnits=m  PxTorqueActuationMode=NoTorque  PxMotionActuationMode=ComputedMotion  PxSensePosition=off  PxSenseVelocity=off  PxSenseAcceleration=off  PxSenseTorqueForce=off  PxSenseLowerLimitTorqueForce=off  PxSenseUpperLimitTorqueForce=off  PyPositionTargetSpecify=on  PyPositionTargetPriority=High  PyPositionTargetValue=rho_It(2)  PyPositionTargetValueUnits=m  PyVelocityTargetSpecify=on  PyVelocityTargetPriority=High  PyVelocityTargetValue=V_It(2)  PyVelocityTargetValueUnits=m/s  PyEquilibriumPosition=0  PyEquilibriumPositionUnits=m  PySpringStiffness=0  PySpringStiffnessUnits=N/m  PyDampingCoefficient=0  PyDampingCoefficientUnits=N/(m/s)  PyLowerLimitSpecify=off  PyLowerLimitBound=-1  PyLowerLimitBoundUnits=m  PyLowerLimitStiffness=1e6  PyLowerLimitStiffnessUnits=N/m  PyLowerLimitDamping=1e3  PyLowerLimitDampingUnits=N/(m/s)  PyLowerLimitTransitionRegionWidth=1e-4  PyLowerLimitTransitionRegionWidthUnits=m  PyUpperLimitSpecify=off  PyUpperLimitBound=1  PyUpperLimitBoundUnits=m  PyUpperLimitStiffness=1e6  PyUpperLimitStiffnessUnits=N/m  PyUpperLimitDamping=1e3  PyUpperLimitDampingUnits=N/(m/s)  PyUpperLimitTransitionRegionWidth=1e-4  PyUpperLimitTransitionRegionWidthUnits=m  PyTorqueActuationMode=NoTorque  PyMotionActuationMode=ComputedMotion  PySensePosition=off  PySenseVelocity=off  PySenseAcceleration=off  PySenseTorqueForce=off  PySenseLowerLimitTorqueForce=off  PySenseUpperLimitTorqueForce=off  PzPositionTargetSpecify=on  PzPositionTargetPriority=High  PzPositionTargetValue=rho_It(3)+sc_size  PzPositionTargetValueUnits=m  PzVelocityTargetSpecify=on  PzVelocityTargetPriority=High  PzVelocityTargetValue=V_It(3)  PzVelocityTargetValueUnits=m/s  PzEquilibriumPosition=0  PzEquilibriumPositionUnits=m  PzSpringStiffness=0  PzSpringStiffnessUnits=N/m  PzDampingCoefficient=0  PzDampingCoefficientUnits=N/(m/s)  PzLowerLimitSpecify=off  PzLowerLimitBound=-1  PzLowerLimitBoundUnits=m  PzLowerLimitStiffness=1e6  PzLowerLimitStiffnessUnits=N/m  PzLowerLimitDamping=1e3  PzLowerLimitDampingUnits=N/(m/s)  PzLowerLimitTransitionRegionWidth=1e-4  PzLowerLimitTransitionRegionWidthUnits=m  PzUpperLimitSpecify=off  PzUpperLimitBound=1  PzUpperLimitBoundUnits=m  PzUpperLimitStiffness=1e6  PzUpperLimitStiffnessUnits=N/m  PzUpperLimitDamping=1e3  PzUpperLimitDampingUnits=N/(m/s)  PzUpperLimitTransitionRegionWidth=1e-4  PzUpperLimitTransitionRegionWidthUnits=m  PzTorqueActuationMode=NoTorque  PzMotionActuationMode=ComputedMotion  PzSensePosition=off  PzSenseVelocity=off  PzSenseAcceleration=off  PzSenseTorqueForce=off  PzSenseLowerLimitTorqueForce=off  PzSenseUpperLimitTorqueForce=off  SphPositionTargetSpecify=on  SphPositionTargetPriority=High  SphPositionTargetRotationMethod=RotationSequence  SphPositionTargetFollAlignAxisA=+X  SphPositionTargetBaseAlignAxisA=+Y  SphPositionTargetFollAlignAxisB=+Y  SphPositionTargetBaseAlignAxisB=+Z  SphPositionTargetRotationStandardAxis=+Z  SphPositionTargetRotationAngle=0.0  SphPositionTargetRotationAngleUnits=deg  SphPositionTargetRotationArbitraryAxis=[0 0 1]  SphPositionTargetRotationSequenceAxes=FollowerAxes  SphPositionTargetRotationSequence=XYZ  SphPositionTargetRotationSequenceAngles=[0 0 0]  SphPositionTargetRotationSequenceAnglesUnits=rad  SphPositionTargetRotationMatrix=[1 0 0; 0 1 0; 0 0 1]  SphPositionTargetQuaternion=[1 0 0 0]  SphVelocityTargetSpecify=on  SphVelocityTargetPriority=High  SphVelocityTargetValue=w_t  SphVelocityTargetValueUnits=rad/s  SphVelocityTargetInFollowerFrame=off  SphEqPosRotationMethod=None  SphEqPosFollAlignAxisA=+X  SphEqPosBaseAlignAxisA=+Y  SphEqPosFollAlignAxisB=+Y  SphEqPosBaseAlignAxisB=+Z  SphEqPosRotationStandardAxis=+Z  SphEqPosRotationAngle=0.0  SphEqPosRotationAngleUnits=deg  SphEqPosRotationArbitraryAxis=[0 0 1]  SphEqPosRotationSequenceAxes=FollowerAxes  SphEqPosRotationSequence=XYX  SphEqPosRotationSequenceAngles=[0 0 0]  SphEqPosRotationSequenceAnglesUnits=deg  SphEqPosRotationMatrix=[1 0 0; 0 1 0; 0 0 1]  SphEqPosQuaternion=[1 0 0 0]  SphSpringStiffness=0  SphSpringStiffnessUnits=N*m/deg  SphDampingCoefficient=0  SphDampingCoefficientUnits=N*m/(deg/s)  SphLowerLimitSpecify=off  SphLowerLimitBound=15  SphLowerLimitBoundUnits=deg  SphLowerLimitStiffness=1e4  SphLowerLimitStiffnessUnits=N*m/deg  SphLowerLimitDamping=10  SphLowerLimitDampingUnits=N*m/(deg/s)  SphLowerLimitTransitionRegionWidth=0.1  SphLowerLimitTransitionRegionWidthUnits=deg  SphUpperLimitSpecify=off  SphUpperLimitBound=45  SphUpperLimitBoundUnits=deg  SphUpperLimitStiffness=1e4  SphUpperLimitStiffnessUnits=N*m/deg  SphUpperLimitDamping=10  SphUpperLimitDampingUnits=N*m/(deg/s)  SphUpperLimitTransitionRegionWidth=0.1  SphUpperLimitTransitionRegionWidthUnits=deg  SphTorqueActuationMode=NoTorque  SphActuateTorqueX=off  SphActuateTorqueY=off  SphActuateTorqueZ=off  SphActuateTorque=off  SphActuationFrame=BaseFrame  SphSensePosition=off  SphSenseVelocityX=off  SphSenseVelocityY=off  SphSenseVelocityZ=off  SphSenseVelocity=off  SphSenseAccelerationX=off  SphSenseAccelerationY=off  SphSenseAccelerationZ=off  SphSenseAcceleration=off  SphSenseLowerLimitTorqueMag=off  SphSenseUpperLimitTorqueMag=off  SphSensingFrame=BaseFrame
  Base Sensing2 : sm_lib/Frames and Transforms/Transform Sensor  MeasurementFrame=NonRotatingBase  RotationSequence=XYZ  SenseAngle=off  SenseAxis=off  SenseQ=off  SenseR=on  SenseRotationSequence=off  SenseOmegaX=on  SenseOmegaY=on  SenseOmegaZ=on  SenseOmega=off  SenseQDot=off  SenseRDot=off  SenseRotationSequenceDot=off  SenseAlphaX=off  SenseAlphaY=off  SenseAlphaZ=off  SenseAlpha=off  SenseQDDot=off  SenseRDDot=off  SenseX=on  SenseY=on  SenseZ=on  SenseXYZ=off  SenseRad=off  SenseAzim=off  SenseDist=off  SenseInc=off  SenseXDot=on  SenseYDot=on  SenseZDot=on  SenseXYZDot=off  SenseRadDot=off  SenseAzimDot=off  SenseDistDot=off  SenseIncDot=off  SenseXDDot=off  SenseYDDot=off  SenseZDDot=off  SenseXYZDDot=off  SenseRadDDot=off  SenseAzimDDot=off  SenseDistDDot=off  SenseIncDDot=off
  Coordinate Transformation Conversion1 : robotcorelib/Coordinate Transformation Conversion  InputRepresentation=Rotation Matrix  InputEulerSequence=ZYX  ShowTrVecInputPort=on  OutputRepresentation=Homogeneous Transformation  OutputEulerSequence=ZYX  ShowTrVecOutputPort=on  SimulateUsing=Interpreted execution
  Mux2 : Mux  Inputs=6
  Mux8 : Mux  Inputs=3
  PS-Simulink Converter{6..8,13,18..19,23..26} (10 alike) : nesl_utility/PS-Simulink Converter  PhysicalDomain=network_engine_domain  SubClassName=ps_output  LeftPortType=input  RightPortType=output  PseudoPeriodic=off  Frequencies=[]  VectorFormat=1-D array  Unit=inherit  AffineConversion=off
  Scope : Scope
  Scope1 : Scope
  Target : sm_lib/Body Elements/Brick Solid  BrickDimensions=[0.02, 0.02, 0.02]  BrickDimensionsUnits=m  ExportEntireGeometry=off  InertiaType=Custom  BasedOnType=Mass  Density=1000  DensityUnits=kg/m^3  Mass=10  MassUnits=kg  CenterOfMass=[0 0 0]  CenterOfMassUnits=m  MomentsOfInertia=[M_t(4,4) M_t(5,5) M_t(6,6)]  MomentsOfInertiaUnits=kg*m^2  ProductsOfInertia=[0 0 0]  ProductsOfInertiaUnits=kg*m^2  GraphicType=Marker  MarkerShape=Sphere  MarkerSize=10  GraphicVisPropType=SimpleVisualProperties  GraphicDiffuseColor=[1.0 0.0 0.0]  GraphicOpacity=0.7  GraphicSpecularColor=[0.5 0.5 0.5 1.0]  GraphicAmbientColor=[0.15 0.15 0.15 1.0]  GraphicEmissiveColor=[0.0 0.0 0.0 1.0]  GraphicShininess=75  DoExposeReferenceFrame=on  SerializedFrames=<Frames><Frame><Id>Frame1</Id><Value><Name>F1</Name><Origin><Source>GeometricFeature</Source><FeatureName>-x -y -z point</FeatureName></Origin><PrimaryAxis><DefinedDirection>+Z</DefinedDirection><Source>ReferenceFrame</Source><SourceDirection>+Z</SourceDirection><FeatureName></FeatureName></PrimaryAxis><SecondaryAxis><DefinedDirection>+X</DefinedDirection><Source>ReferenceFrame</Source><SourceDirection>+X</SourceDirection><FeatureName></FeatureName></SecondaryAxis></Value></Frame></Frames>
  Conn1 : PMIOPort  Side=Left
  g_I_target : Outport
  V_It_t : Outport  Port=2
  wires:
  PS-Simulink Converter13/1 -> Mux8/3
  Coordinate Transformation Conversion1/1 -> g_I_target/1
  PS-Simulink Converter7/1 -> Mux8/1
  PS-Simulink Converter6/1 -> Coordinate Transformation Conversion1/1
  PS-Simulink Converter8/1 -> Mux8/2
  Mux8/1 -> Scope/1, Coordinate Transformation Conversion1/2
  PS-Simulink Converter24/1 -> Mux2/4
  PS-Simulink Converter18/1 -> Mux2/2
  PS-Simulink Converter25/1 -> Mux2/5
  Mux2/1 -> Scope1/1, V_It_t/1
  PS-Simulink Converter19/1 -> Mux2/1
  PS-Simulink Converter23/1 -> Mux2/3
  PS-Simulink Converter26/1 -> Mux2/6
  connections:
  Base Sensing2/RConn2 -- PS-Simulink Converter6/LConn1
  Base Sensing2/RConn3 -- PS-Simulink Converter24/LConn1
  6-DOF Joint1/LConn1 -- Base Sensing2/LConn1 -- Conn1/RConn1
  Base Sensing2/RConn5 -- PS-Simulink Converter26/LConn1
  Base Sensing2/RConn4 -- PS-Simulink Converter25/LConn1
  Base Sensing2/RConn6 -- PS-Simulink Converter7/LConn1
  Base Sensing2/RConn7 -- PS-Simulink Converter8/LConn1
  Base Sensing2/RConn8 -- PS-Simulink Converter13/LConn1
  Base Sensing2/RConn9 -- PS-Simulink Converter19/LConn1
  Base Sensing2/RConn10 -- PS-Simulink Converter18/LConn1
  Base Sensing2/RConn11 -- PS-Simulink Converter23/LConn1
  6-DOF Joint1/RConn1 -- Target/RConn1 -- Base Sensing2/RConn1
